simulink model "Copy_of_cascade_ref_model"  (R2020a)
settings: Solver=FixedStepDiscrete  StartTime=0.0  StopTime=10.0  RelTol=1e-3
settings Model: Creator=Prateek  LastModifiedBy=Prateek
settings DataIOCC: SaveOutput=off  SaveTime=off

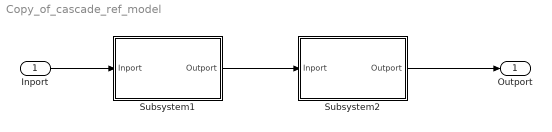
== system Copy_of_cascade_ref_model ==
  Inport : Inport  OutDataTypeStr=double  PortDimensions=1  SampleTime=0
  Subsystem1 : Subsystem
  Subsystem2 : Subsystem
  Outport : Outport  OutDataTypeStr=double  PortDimensions=1  SampleTime=0
  wires:
  Subsystem1/1(Outport) -> Subsystem2/1(Inport)
  Inport/1 -> Subsystem1/1(Inport)
  Subsystem2/1(Outport) -> Outport/1

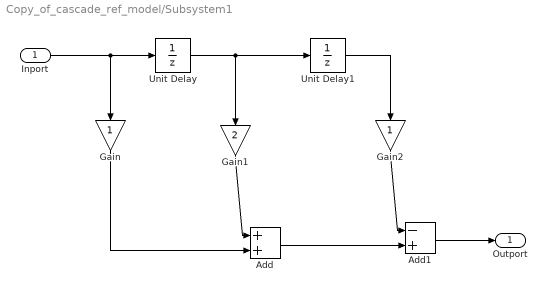
== system Copy_of_cascade_ref_model/Subsystem1 ==
  Inport : Inport
  Add : Sum
  Add1 : Sum  Inputs=-+
  Gain : Gain
  Gain1 : Gain  Gain=2
  Gain2 : Gain
  Unit Delay : UnitDelay  SampleTime=-1  HasFrameUpgradeWarning=on
  Unit Delay1 : UnitDelay  SampleTime=-1  HasFrameUpgradeWarning=on
  Outport : Outport
  wires:
  Gain1/1 -> Add/1
  Add/1 -> Add1/2
  Gain/1 -> Add/2
  Unit Delay1/1 -> Gain2/1
  Gain2/1 -> Add1/1
  Inport/1 -> Unit Delay/1, Gain/1
  Unit Delay/1 -> Gain1/1, Unit Delay1/1
  Add1/1 -> Outport/1

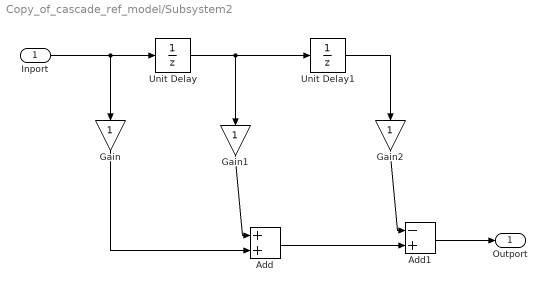
== system Copy_of_cascade_ref_model/Subsystem2 ==
  Inport : Inport
  Add : Sum
  Add1 : Sum  Inputs=-+
  Gain : Gain
  Gain1 : Gain
  Gain2 : Gain
  Unit Delay : UnitDelay  SampleTime=-1  HasFrameUpgradeWarning=on
  Unit Delay1 : UnitDelay  SampleTime=-1  HasFrameUpgradeWarning=on
  Outport : Outport
  wires:
  Gain1/1 -> Add/1
  Add/1 -> Add1/2
  Gain/1 -> Add/2
  Unit Delay1/1 -> Gain2/1
  Gain2/1 -> Add1/1
  Inport/1 -> Unit Delay/1, Gain/1
  Unit Delay/1 -> Gain1/1, Unit Delay1/1
  Add1/1 -> Outport/1
